simulink model "MotorModule"  (R2021a)
settings: Solver=FixedStepAuto  StartTime=0.0  StopTime=inf  FixedStep=0.002  RelTol=1e-3  EnableMultiTasking=on
libraries: can_bus_multi x1
settings Model: Creator=ASUS  LastModifiedBy=ASUS
settings SolverCC: PositivePriorityOrder=on
settings OptimizationCC: EnhancedBackFolding=on  PassReuseOutputArgsAs=Individual arguments  ZeroExternalMemoryAtStartup=off  ZeroInternalMemoryAtStartup=off  MaxStackSize=64  OptimizeBlockOrder=speed  DifferentSizesBufferReuse=on  OptimizationCustomize=off  EfficientTunableParamExpr=on
settings DebuggingCC: ParameterTunabilityLossMsg=error
settings HardwareCC: ProdBitPerPointer=32  ProdBitPerSizeT=32  ProdBitPerPtrDiffT=32  ProdLargestAtomicInteger=Long  ProdLargestAtomicFloat=Double  ProdWordSize=32  ProdLongLongMode=on  ProdHWDeviceType=ARM Compatible->ARM Cortex
settings RTWCC: SystemTargetFile=ert.tlc  HardwareBoard=Raspberry Pi  TLCOptions="-aInlineSetEventsForThisBaseRateFcn=TLC_FALSE -aSuppressMultiTaskScheduler=TLC_FALSE  -aRateBasedStepFcn=0"  TemplateMakefile=ert_default_tmf  Toolchain=GNU GCC Embedded Linux  BuildConfiguration=Specify  TargetLang=C++
settings CodeAppCC: ForceParamTrailComments=on  IgnoreCustomStorageClasses=off  OperatorAnnotations=on  SimulinkDataObjDesc=on  SFDataObjDesc=on  InsertBlockDesc=on
settings ERTTargetCC: TargetLangStandard=C++03 (ISO)  SupportContinuousTime=on  SupportVariableSizeSignals=on  ExtModeTransport=2  ExtModeStaticAlloc=on  ExtModeMexFile=ext_xcp  ExtModeIntrfLevel=Level2 - Open  RootIOFormat=Structure reference

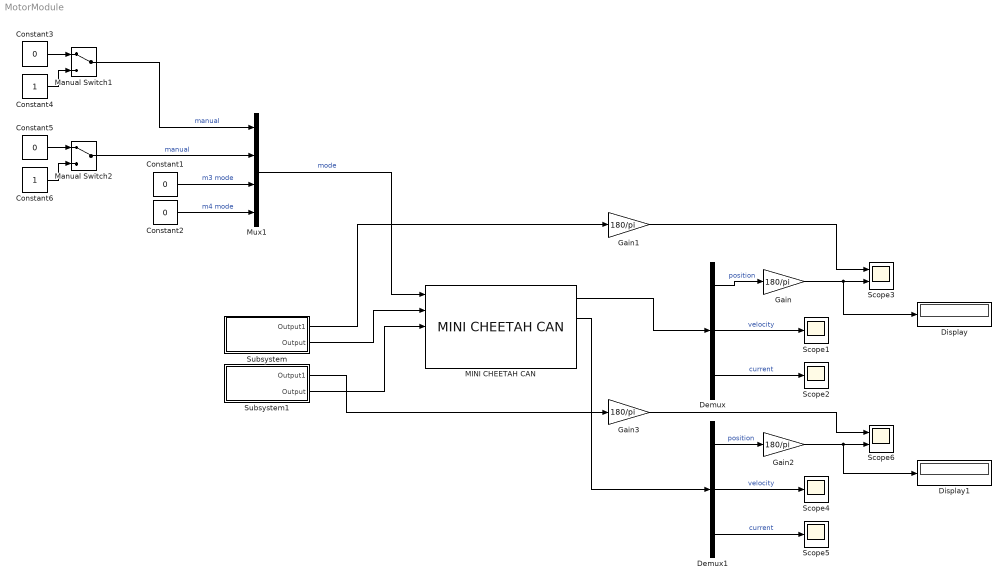
== system MotorModule ==
  Constant{1..3,5} (4 alike) : Constant  Value=0
  Constant4 : Constant
  Constant6 : Constant
  Demux : Demux  Outputs=3
  Demux1 : Demux  Outputs=3
  Display : Display
  Display1 : Display
  Gain{,1..3} (4 alike) : Gain  Gain=180/pi
  MINI CHEETAH CAN : can_bus_multi/MINI CHEETAH CAN  PAR_PORT_NUM=can0  PAR_SAFE=on  PAR_DEV_NUM=2  PAR_SMPLT=0.002
      settings: SourceProductName=CAN Bus Multi
  Manual Switch1 : ManualSwitch
  Manual Switch2 : ManualSwitch
  Mux1 : Mux
  Scope{1..2,4..5} (4 alike) : Scope
  Scope3 : Scope  NumInputPorts=2
  Scope6 : Scope  NumInputPorts=2
  Subsystem : Subsystem
  Subsystem1 : Subsystem
  wires:
  Subsystem/2(Output) -> MINI CHEETAH CAN/2
  Mux1/1 -> MINI CHEETAH CAN/1  "mode"
  Constant3/1 -> Manual Switch1/1
  Manual Switch1/1 -> Mux1/1  "manual"
  Constant4/1 -> Manual Switch1/2
  Constant1/1 -> Mux1/3  "m3 mode"
  Constant2/1 -> Mux1/4  "m4 mode"
  Demux/2 -> Scope1/1  "velocity"
  MINI CHEETAH CAN/1 -> Demux/1
  Demux/3 -> Scope2/1  "current"
  Demux/1 -> Gain/1  "position"
  Gain/1 -> Display/1, Scope3/2
  Gain1/1 -> Scope3/1
  Subsystem/1(Output1) -> Gain1/1
  Subsystem1/2(Output) -> MINI CHEETAH CAN/3
  MINI CHEETAH CAN/2 -> Demux1/1
  Demux1/3 -> Scope5/1  "current"
  Demux1/2 -> Scope4/1  "velocity"
  Demux1/1 -> Gain2/1  "position"
  Gain2/1 -> Scope6/2, Display1/1
  Gain3/1 -> Scope6/1
  Subsystem1/1(Output1) -> Gain3/1
  Constant5/1 -> Manual Switch2/1
  Constant6/1 -> Manual Switch2/2
  Manual Switch2/1 -> Mux1/2  "manual"

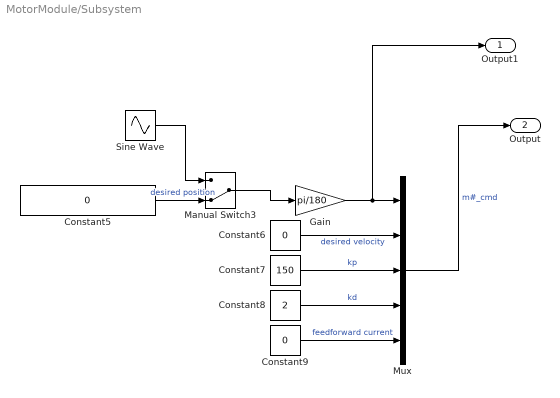
== system MotorModule/Subsystem ==
  Constant5 : Constant  Value=0
  Constant6 : Constant  Value=0
  Constant7 : Constant  Value=150
  Constant8 : Constant  Value=2
  Constant9 : Constant  Value=0
  Gain : Gain  Gain=pi/180
  Manual Switch3 : ManualSwitch  CurrentSetting=0
  Mux : Mux  Inputs=5
  Sine Wave : Sin  Amplitude=20  Frequency=8*pi  SampleTime=0
  Output1 : Outport
  Output : Outport  Port=2
  wires:
  Sine Wave/1 -> Manual Switch3/1
  Constant9/1 -> Mux/5  "feedforward current"
  Constant5/1 -> Manual Switch3/2  "desired position"
  Manual Switch3/1 -> Gain/1
  Constant7/1 -> Mux/3  "kp"
  Gain/1 -> Output1/1, Mux/1
  Mux/1 -> Output/1  "m#_cmd"
  Constant6/1 -> Mux/2  "desired velocity"
  Constant8/1 -> Mux/4  "kd"

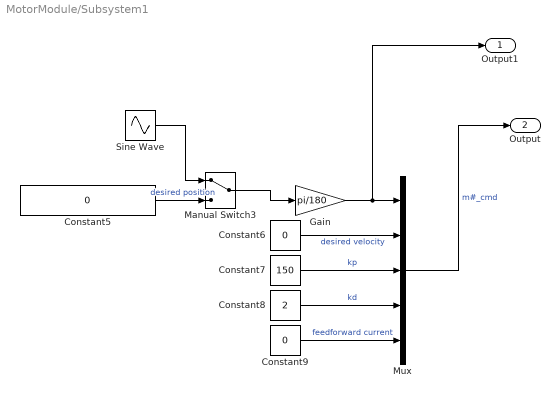
== system MotorModule/Subsystem1 ==
  Constant5 : Constant  Value=0
  Constant6 : Constant  Value=0
  Constant7 : Constant  Value=150
  Constant8 : Constant  Value=2
  Constant9 : Constant  Value=0
  Gain : Gain  Gain=pi/180
  Manual Switch3 : ManualSwitch
  Mux : Mux  Inputs=5
  Sine Wave : Sin  Amplitude=20  Frequency=8*pi  SampleTime=0
  Output1 : Outport
  Output : Outport  Port=2
  wires:
  Sine Wave/1 -> Manual Switch3/1
  Constant9/1 -> Mux/5  "feedforward current"
  Constant5/1 -> Manual Switch3/2  "desired position"
  Manual Switch3/1 -> Gain/1
  Constant7/1 -> Mux/3  "kp"
  Gain/1 -> Output1/1, Mux/1
  Mux/1 -> Output/1  "m#_cmd"
  Constant6/1 -> Mux/2  "desired velocity"
  Constant8/1 -> Mux/4  "kd"
